simulink model "modelo_ARX_indirecto"  (R2015a)
settings: Solver=ode45  StartTime=0.0  StopTime=1000  RelTol=1e-3
values from neighbouring files (symbols this model uses):
  lambda = 1    [generar_prbs.m]    (also in parametros_ident.m = 0.995)
libraries: dspsigops x2
settings Model: Creator=u_labelectro  LastModifiedBy=Luis
settings DebuggingCC: UnderspecifiedInitializationDetection=Classic  MergeDetectMultiDrivingBlocksExec=none  SolverPrmCheckMsg=warning  StateNameClashWarn=warning

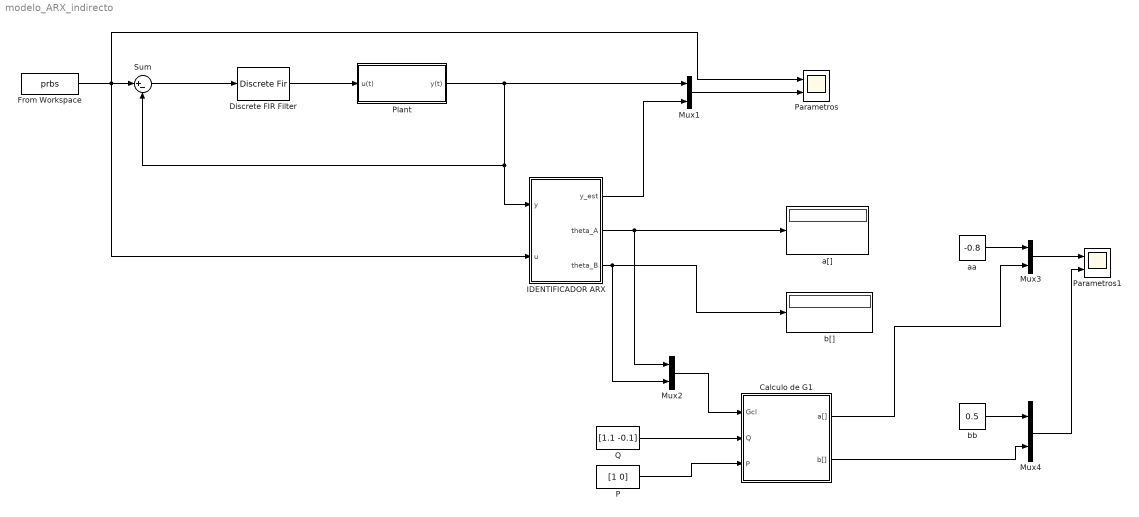
== system modelo_ARX_indirecto ==
  Calculo de G1 : Subsystem
  Discrete FIR Filter : DiscreteFir  Coefficients=[1.1 -0.1]  SampleTime=0.1
  From Workspace : FromWorkspace  VariableName=prbs
  IDENTIFICADOR ARX : Subsystem
  Mux{1..4} (4 alike) : Mux  Inputs=2
  P : Constant  Value=[1 0]
  Parametros : Scope  NumInputPorts=2
      settings: TimeRange=100  YMin=0~-0.5  YMax=5~10
  Parametros1 : Scope  NumInputPorts=2
      settings: YMin=-5~-5  YMax=5~5
  Plant : Subsystem
  Q : Constant  Value=[1.1 -0.1]
  Sum : Sum  Inputs=|+-
  a[] : Display
  aa : Constant  Value=-0.8
  b[] : Display
  bb : Constant  Value=0.5
  wires:
  Sum/1 -> Discrete FIR Filter/1
  Discrete FIR Filter/1 -> Plant/1(u(t))
  Plant/1(y(t)) -> IDENTIFICADOR ARX/1(y), Sum/2, Mux1/1
  Mux1/1 -> Parametros/2
  IDENTIFICADOR ARX/2(theta_A) -> Mux2/1, a[]/1
  IDENTIFICADOR ARX/3(theta_B) -> Mux2/2, b[]/1
  IDENTIFICADOR ARX/1(y_est) -> Mux1/2
  Mux2/1 -> Calculo de G1/1(Gcl)
  aa/1 -> Mux3/1
  Calculo de G1/1(a[]) -> Mux3/2
  bb/1 -> Mux4/1
  Calculo de G1/2(b[]) -> Mux4/2
  Mux3/1 -> Parametros1/1
  Mux4/1 -> Parametros1/2
  Q/1 -> Calculo de G1/2(Q)
  P/1 -> Calculo de G1/3(P)
  From Workspace/1 -> IDENTIFICADOR ARX/2(u), Parametros/1, Sum/1

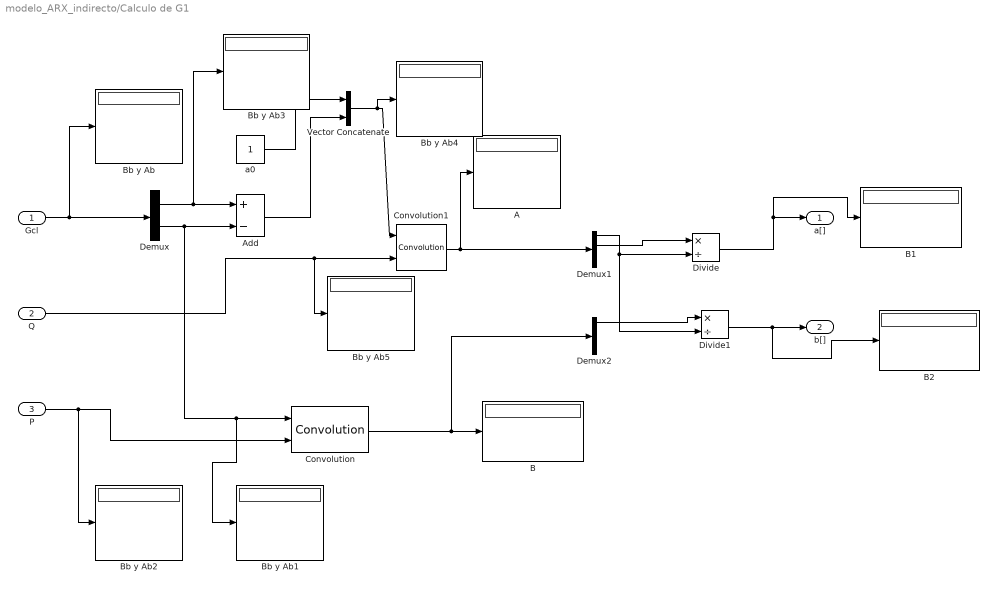
== system modelo_ARX_indirecto/Calculo de G1 ==
  Gcl : Inport
  Q : Inport  Port=2
  P : Inport  Port=3
  A : Display
  Add : Sum  Inputs=+-
  B : Display
  B1 : Display
  B2 : Display
  Bb y Ab{,1..5} (6 alike) : Display
  Convolution : dspsigops/Convolution  domain=Time  outputDataTypeStr=Inherit: Same as accumulator  outputLastDataTypeStr=Inherit: Same as accumulator  outputMin=[]  outputMax=[]  roundingMode=Floor  overflowMode=off
  Convolution1 : dspsigops/Convolution  domain=Time  outputDataTypeStr=Inherit: Same as accumulator  outputLastDataTypeStr=Inherit: Same as accumulator  outputMin=[]  outputMax=[]  roundingMode=Floor  overflowMode=off
  Demux : Demux  Outputs=2
  Demux1 : Demux
  Demux2 : Demux  Outputs=3
  Divide : Product  Inputs=*/
  Divide1 : Product  Inputs=*/
  Vector Concatenate : Concatenate
  a0 : Constant
  a[] : Outport
  b[] : Outport  Port=2
  wires:
  Gcl/1 -> Bb y Ab/1, Demux/1
  a0/1 -> Vector Concatenate/1
  Divide/1 -> B1/1, a[]/1
  Divide1/1 -> B2/1, b[]/1
  Vector Concatenate/1 -> Bb y Ab4/1, Convolution1/1
  Q/1 -> Bb y Ab5/1, Convolution1/2
  P/1 -> Bb y Ab2/1, Convolution/2
  Convolution/1 -> Demux2/1, B/1
  Convolution1/1 -> A/1, Demux1/1
  Demux1/2 -> Divide/1
  Demux1/1 -> Divide1/2, Divide/2
  Demux2/1 -> Divide1/1
  Add/1 -> Vector Concatenate/2
  Demux/1 -> Bb y Ab3/1, Add/1
  Demux/2 -> Bb y Ab1/1, Convolution/1, Add/2

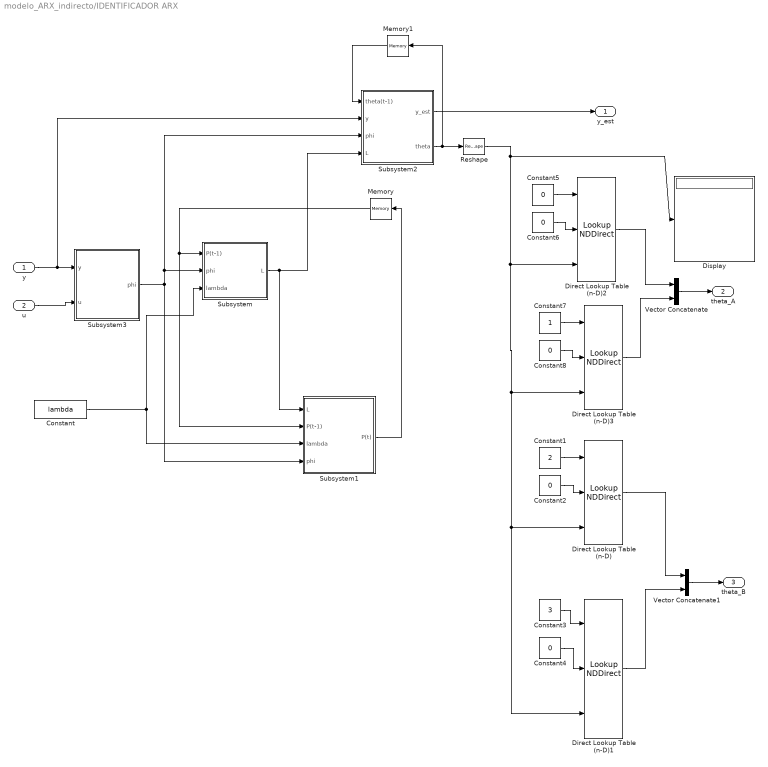
== system modelo_ARX_indirecto/IDENTIFICADOR ARX ==
  y : Inport
  u : Inport  Port=2
  Constant : Constant  Value=lambda
  Constant1 : Constant  Value=2
  Constant{2,4..6,8} (5 alike) : Constant  Value=0
  Constant3 : Constant  Value=3
  Constant7 : Constant
  Direct Lookup Table (n-D){,1..3} (4 alike) : LookupNDDirect  TableIsInput=on  Table=[4 5 ;16 19 ]  DiagnosticForOutOfRangeInput=Error
  Display : Display
  Memory : Memory  X0=1e6*eye(4)
  Memory1 : Memory
  Reshape : Reshape  OutputDimensionality=Column vector (2-D)
  Subsystem : Subsystem
  Subsystem1 : Subsystem
  Subsystem2 : Subsystem
  Subsystem3 : Subsystem
  Vector Concatenate : Concatenate
  Vector Concatenate1 : Concatenate
  y_est : Outport
  theta_A : Outport  Port=2
  theta_B : Outport  Port=3
  wires:
  y/1 -> Subsystem2/2(y), Subsystem3/1(y)
  Subsystem3/1(phi) -> Subsystem1/4(phi), Subsystem2/3(phi), Subsystem/2(phi)
  Subsystem/1(L) -> Subsystem1/1(L), Subsystem2/4(L)
  u/1 -> Subsystem3/2(u)
  Constant/1 -> Subsystem1/3(lambda), Subsystem/3(lambda)
  Subsystem1/1(P(t)) -> Memory/1
  Memory/1 -> Subsystem1/2(P(t-1)), Subsystem/1(P(t-1))
  Subsystem2/1(y_est) -> y_est/1
  Subsystem2/2(theta) -> Reshape/1, Memory1/1
  Memory1/1 -> Subsystem2/1(theta(t-1))
  Constant4/1 -> Direct Lookup Table (n-D)1/2
  Constant3/1 -> Direct Lookup Table (n-D)1/1
  Constant2/1 -> Direct Lookup Table (n-D)/2
  Constant1/1 -> Direct Lookup Table (n-D)/1
  Reshape/1 -> Direct Lookup Table (n-D)2/3, Direct Lookup Table (n-D)3/3, Direct Lookup Table (n-D)1/3, Direct Lookup Table (n-D)/3, Display/1
  Constant6/1 -> Direct Lookup Table (n-D)2/2
  Constant5/1 -> Direct Lookup Table (n-D)2/1
  Constant8/1 -> Direct Lookup Table (n-D)3/2
  Constant7/1 -> Direct Lookup Table (n-D)3/1
  Direct Lookup Table (n-D)1/1 -> Vector Concatenate1/2
  Direct Lookup Table (n-D)/1 -> Vector Concatenate1/1
  Vector Concatenate1/1 -> theta_B/1
  Direct Lookup Table (n-D)3/1 -> Vector Concatenate/2
  Direct Lookup Table (n-D)2/1 -> Vector Concatenate/1
  Vector Concatenate/1 -> theta_A/1

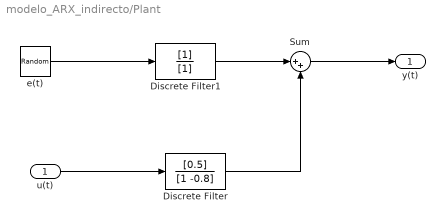
== system modelo_ARX_indirecto/Plant ==
  u(t) : Inport
  Discrete Filter : DiscreteFilter  Numerator=[0.5]  Denominator=[1 -0.8]
  Discrete Filter1 : DiscreteFilter  Denominator=[1]  SampleTime=0.1
  Sum : Sum  Inputs=|++
  e(t) : RandomNumber  Variance=0.003
  y(t) : Outport
  wires:
  Discrete Filter/1 -> Sum/2
  Discrete Filter1/1 -> Sum/1
  Sum/1 -> y(t)/1
  u(t)/1 -> Discrete Filter/1
  e(t)/1 -> Discrete Filter1/1

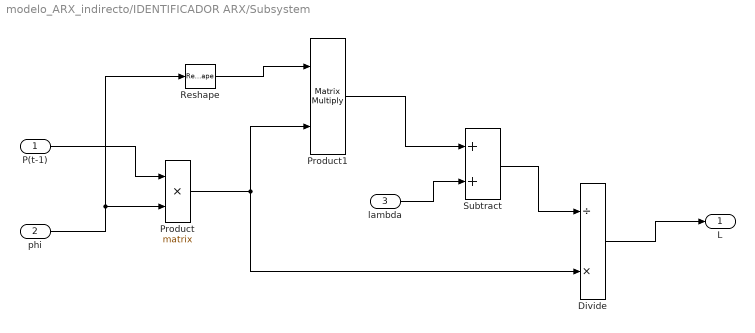
== system modelo_ARX_indirecto/IDENTIFICADOR ARX/Subsystem ==
  P(t-1) : Inport
  phi : Inport  Port=2
  lambda : Inport  Port=3
  Divide : Product  Inputs=/*
  Product : Product  Multiplication=Matrix(*)
  Product1 : Product  Multiplication=Matrix(*)
  Reshape : Reshape  OutputDimensionality=Row vector (2-D)
  Subtract : Sum
  L : Outport
  wires:
  Divide/1 -> L/1
  Subtract/1 -> Divide/1
  phi/1 -> Reshape/1, Product/2
  Reshape/1 -> Product1/1
  Product1/1 -> Subtract/1
  lambda/1 -> Subtract/2
  Product/1 -> Product1/2, Divide/2
  P(t-1)/1 -> Product/1

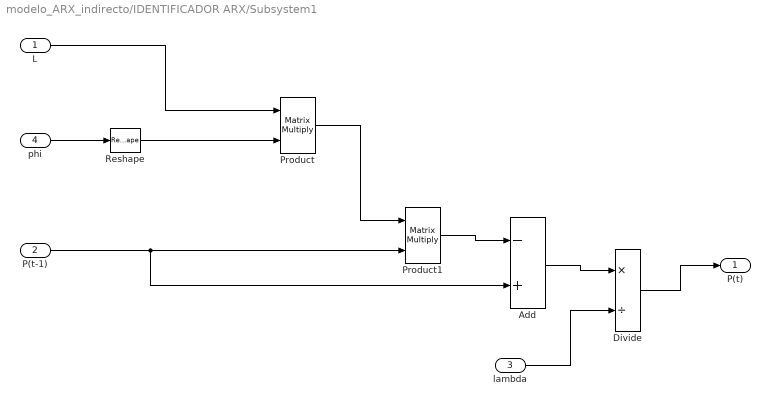
== system modelo_ARX_indirecto/IDENTIFICADOR ARX/Subsystem1 ==
  L : Inport
  P(t-1) : Inport  Port=2
  lambda : Inport  Port=3
  phi : Inport  Port=4
  Add : Sum  Inputs=-+
  Divide : Product  Inputs=*/
  Product : Product  Multiplication=Matrix(*)
  Product1 : Product  Multiplication=Matrix(*)
  Reshape : Reshape  OutputDimensionality=Row vector (2-D)
  P(t) : Outport
  wires:
  L/1 -> Product/1
  phi/1 -> Reshape/1
  Reshape/1 -> Product/2
  Product/1 -> Product1/1
  P(t-1)/1 -> Add/2, Product1/2
  Product1/1 -> Add/1
  Add/1 -> Divide/1
  Divide/1 -> P(t)/1
  lambda/1 -> Divide/2

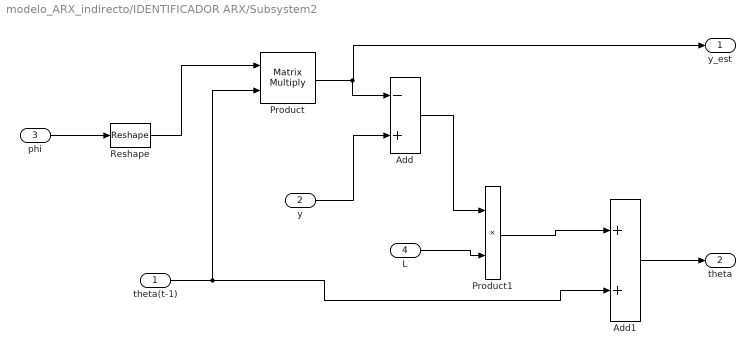
== system modelo_ARX_indirecto/IDENTIFICADOR ARX/Subsystem2 ==
  theta(t-1) : Inport
  y : Inport  Port=2
  phi : Inport  Port=3
  L : Inport  Port=4
  Add : Sum  Inputs=-+
  Add1 : Sum
  Product : Product  Multiplication=Matrix(*)
  Product1 : Product
  Reshape : Reshape  OutputDimensionality=Row vector (2-D)
  y_est : Outport
  theta : Outport  Port=2
  wires:
  Product/1 -> Add/1, y_est/1
  y/1 -> Add/2
  L/1 -> Product1/2
  Add/1 -> Product1/1
  Product1/1 -> Add1/1
  Add1/1 -> theta/1
  theta(t-1)/1 -> Product/2, Add1/2
  Reshape/1 -> Product/1
  phi/1 -> Reshape/1

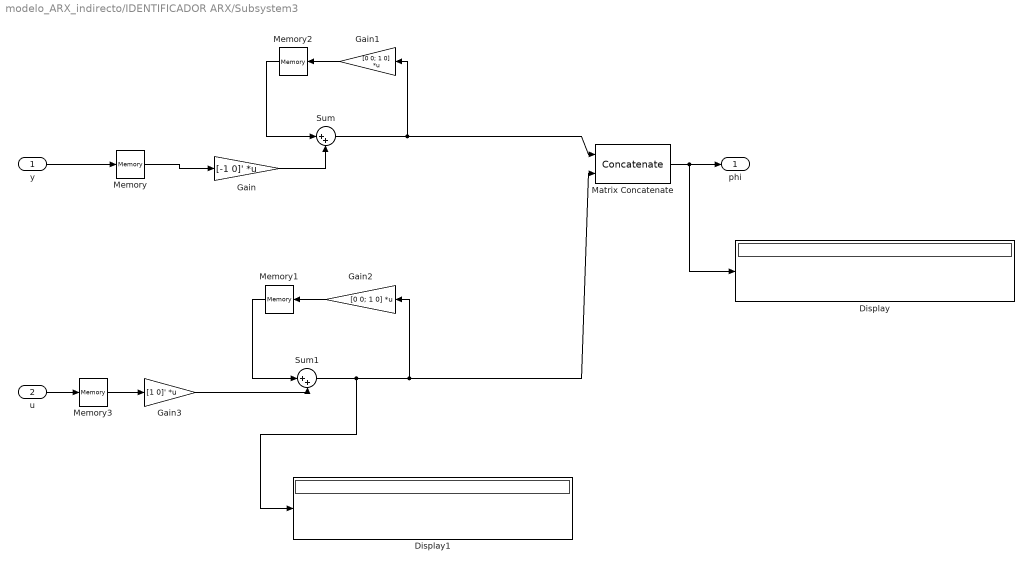
== system modelo_ARX_indirecto/IDENTIFICADOR ARX/Subsystem3 ==
  y : Inport
  u : Inport  Port=2
  Display : Display
  Display1 : Display
  Gain : Gain  Gain=[-1 0]'  Multiplication=Matrix(K*u)
  Gain1 : Gain  Gain=[0 0; 1 0]  Multiplication=Matrix(K*u)
  Gain2 : Gain  Gain=[0 0; 1 0]  Multiplication=Matrix(K*u)
  Gain3 : Gain  Gain=[1 0]'  Multiplication=Matrix(K*u)
  Matrix Concatenate : Concatenate  Mode=Multidimensional array
  Memory{,1..3} (4 alike) : Memory
  Sum : Sum  Inputs=|++
  Sum1 : Sum  Inputs=|++
  phi : Outport
  wires:
  Gain1/1 -> Memory2/1
  Memory2/1 -> Sum/1
  Gain/1 -> Sum/2
  Memory/1 -> Gain/1
  y/1 -> Memory/1
  Gain2/1 -> Memory1/1
  Gain3/1 -> Sum1/2
  Memory1/1 -> Sum1/1
  Sum/1 -> Matrix Concatenate/1, Gain1/1
  Sum1/1 -> Display1/1, Gain2/1, Matrix Concatenate/2
  u/1 -> Memory3/1
  Memory3/1 -> Gain3/1
  Matrix Concatenate/1 -> Display/1, phi/1
